simulink model "pociag"  (R2018b)
settings: Solver=VariableStepAuto  StartTime=0.0  StopTime=10.0  RelTol=1e-3
settings Model: Creator=bartl  LastModifiedBy=Kasia

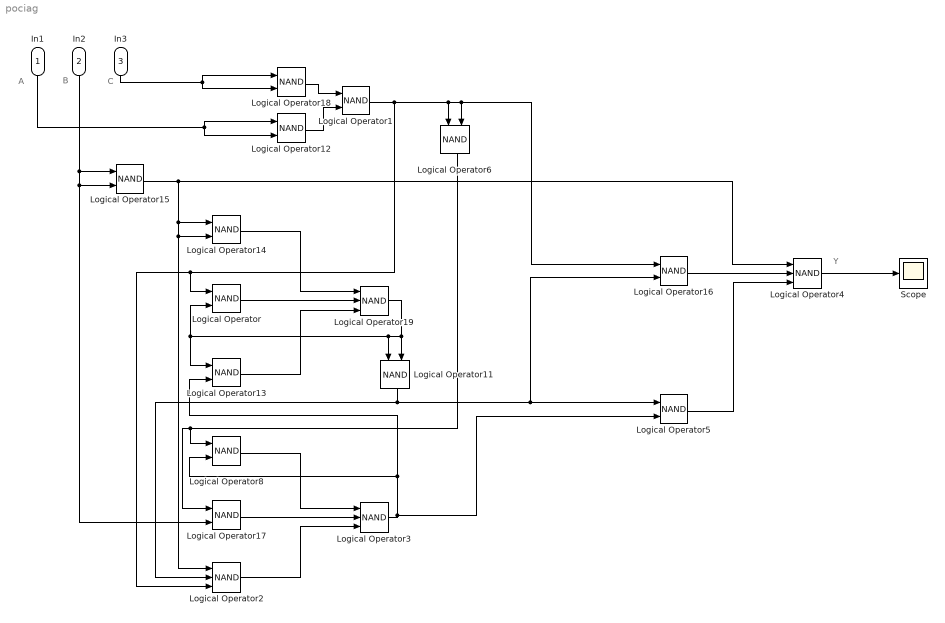
== system pociag ==
  note: Y
  note: C
  note: B
  note: A
  In1 : Inport  OutMin=0  OutMax=0  OutDataTypeStr=boolean
  In2 : Inport  Port=2  OutMin=1  OutMax=1  OutDataTypeStr=boolean
  In3 : Inport  Port=3  OutMin=1  OutMax=1  OutDataTypeStr=boolean
  Logical Operator{,1,5..6,8,11..18} (13 alike) : Logic  Operator=NAND  AllPortsSameDT=off  OutDataTypeStr=boolean
  Logical Operator{2..4,19} (4 alike) : Logic  Operator=NAND  Inputs=3  AllPortsSameDT=off  OutDataTypeStr=boolean
  Scope : Scope
  wires:
  In3/1 -> Logical Operator18/2, Logical Operator18/1
  In1/1 -> Logical Operator12/1, Logical Operator12/2
  Logical Operator18/1 -> Logical Operator1/1
  Logical Operator12/1 -> Logical Operator1/2
  In2/1 -> Logical Operator17/2, Logical Operator15/2, Logical Operator15/1
  Logical Operator15/1 -> Logical Operator2/1, Logical Operator14/2, Logical Operator14/1, Logical Operator4/1
  Logical Operator14/1 -> Logical Operator19/1
  Logical Operator/1 -> Logical Operator19/2
  Logical Operator13/1 -> Logical Operator19/3
  Logical Operator8/1 -> Logical Operator3/1
  Logical Operator17/1 -> Logical Operator3/2
  Logical Operator2/1 -> Logical Operator3/3
  Logical Operator19/1 -> Logical Operator/2, Logical Operator13/1, Logical Operator11/1, Logical Operator11/2
  Logical Operator1/1 -> Logical Operator16/1, Logical Operator6/2, Logical Operator6/1, Logical Operator/1, Logical Operator2/3
  Logical Operator3/1 -> Logical Operator13/2, Logical Operator8/2, Logical Operator5/2
  Logical Operator6/1 -> Logical Operator8/1, Logical Operator17/1
  Logical Operator11/1 -> Logical Operator16/2, Logical Operator5/1, Logical Operator2/2
  Logical Operator4/1 -> Scope/1
  Logical Operator16/1 -> Logical Operator4/2
  Logical Operator5/1 -> Logical Operator4/3
